simulink model "sdm"  (R2024b)
settings: Solver=VariableStepAuto  StartTime=0.0  StopTime=10.0  RelTol=1e-3
values from neighbouring files (symbols this model uses):
  b = 10    [untitled.m]
  F = 1    [untitled.m]    (also in variables_for_parameters.m = 2)
  k = 20    [untitled.m]
  M = 1    [untitled.m]
settings Model: Creator=kavin  LastModifiedBy=kavin

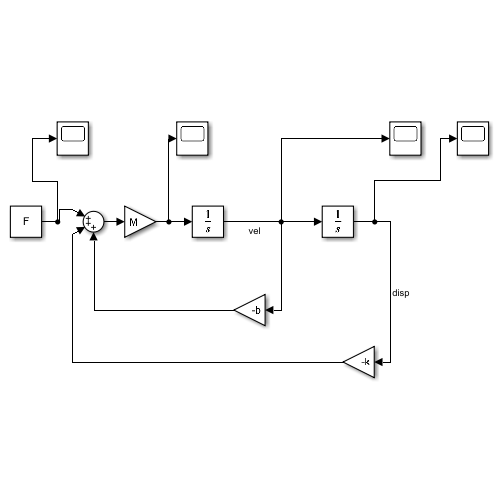
[thumbnail: Simulink's stored preview of the top-level diagram]
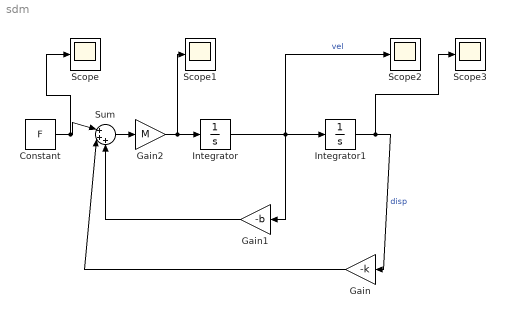
== system sdm ==
  Constant : Constant  Value=F
  Gain : Gain  Gain=-k
  Gain1 : Gain  Gain=-b
  Gain2 : Gain  Gain=M
  Integrator : Integrator
  Integrator1 : Integrator
  Scope{,1..3} (4 alike) : Scope
  Sum : Sum  Inputs=|+++
  wires:
  Integrator/1 -> Scope2/1, Gain1/1, Integrator1/1  "vel"
  Integrator1/1 -> Scope3/1, Gain/1  "disp"
  Constant/1 -> Scope/1, Sum/1
  Gain/1 -> Sum/2
  Gain1/1 -> Sum/3
  Sum/1 -> Gain2/1
  Gain2/1 -> Scope1/1, Integrator/1
